simulink model "zynqRadioHWSWQPSKAD9361AD9364SL"  (R2025a)
settings: Solver=FixedStepDiscrete  StartTime=0.0  StopTime=0.5  RelTol=1e-3
PreLoadFcn:
  | setTxBurstLength = 10000;
  | txtmsg = ['Zynq radio HW/SW Co-design ÞÞÞÞ']; % Use only printable characters
  | 
  | %------------------------------------------------------------------------------------------------------
  | if ~isequal(size(txtmsg),[1 31])
  |     error('txtmsg must contain 31 characters');
  | end
  | 
  | [dataBits,msg] = zynqRadioHWSWQPSKgenHelloworldMsg(20); % generate 20 msgs for LUT
  | msgLUT = uint8(msg);
  | dataBitsLUT = dataBits(:);
  | Rsym                = 10e3;%1.92e6;
  | Config = zynqRadioHWSWQPSKTxRxParameters;
  | fs = Rsym*Config.SamplesPerSymbol;
  | word = [txtmsg newline];  % append a new line character to txtmsg
  | 
  | % The highest clock rate is 16 times the message character rate.
  | % As the message characters are fed at highest clock to FPGA
  | % repeat each character 16 times to maintain the message rate.
  | word = repelem(word.',16,1);
  | repeatTimes = ceil(setTxBurstLength/length(word));
  | inpData = complex(repmat(uint8(word),repeatTimes,1));
  | inUseTxBurstLength = length(inpData);
PostLoadFcn:
  | hScopeConfig = get_param([gcs '/HDL_QPSK/QPSK Tx Channel QPSK Rx/QPSK Rx/Frequency and Time Synchronizer/Symbol Synchronizer/No HDL/QPSK Receiver Eye Diagram'],'ScopeConfiguration');
  | hScopeConfig.OpenAtSimulationStart = false;
  | hScopeConfig.Visible = false;
  | clear hScopeConfig
InitFcn:
  | setTxBurstLength = 10000;
  | txtmsg = ['Zynq radio HW/SW Co-design ÞÞÞÞ']; % Use only printable characters
  | 
  | %------------------------------------------------------------------------------------------------------
  | if ~isequal(size(txtmsg),[1 31])
  |     error('txtmsg must contain 31 characters');
  | end
  | 
  | [dataBits,msg] = zynqRadioHWSWQPSKgenHelloworldMsg(20); % generate 20 msgs for LUT
  | msgLUT = uint8(msg);
  | dataBitsLUT = dataBits(:);
  | Rsym                = 10e3;%1.92e6;
  | Config = zynqRadioHWSWQPSKTxRxParameters;
  | fs = Rsym*Config.SamplesPerSymbol;
  | word = [txtmsg newline];  % append a new line character to txtmsg
  | 
  | % The highest clock rate is 16 times the message character rate.
  | % As the message characters are fed at highest clock to FPGA
  | % repeat each character 16 times to maintain the message rate.
  | word = repelem(word.',16,1);
  | repeatTimes = ceil(setTxBurstLength/length(word));
  | inpData = complex(repmat(uint8(word),repeatTimes,1));
  | inUseTxBurstLength = length(inpData);
  | 
  | Config.Preamble = logical(zeros(0,1))
undefined symbols (not defined in the file or in its folder): Add, dspblkCoreblockFVToolHelper, gcbh, gse_genframes, Shift
libraries: hdlsllib x144, simulink x37, dsphdlsigops2 x3, dsphdlfiltering2 x3, whdlutilities x3, dsphdlxfrm2 x2, dsphdlmathfun2 x2, commdigbbndpm3 x2, sdrzblksprivate x1
(part 3 of 6)

== system zynqRadioHWSWQPSKAD9361AD9364SL/HDL_QPSK/QPSK Tx Channel QPSK Rx/QPSK Rx/Frequency and Time Synchronizer/Symbol Synchronizer ==
  dataIn : Inport
  validIn : Inport  Port=2
  Data Type Conversion4 : DataTypeConversion  OutDataTypeStr=fixdt(1,16,14)  SaturateOnIntegerOverflow=off  RndMeth=Floor
  Delay{1..4,6,8..9} (7 alike) : Delay  DelayLength=1
  Delay5 : Delay  DelayLength=12
  Delay7 : Delay  DelayLength=12
  Gardner TED : Subsystem
  Integer Delay{1..4} (4 alike) : Delay  DelayLength=1
  Interpolation Control : MATLAB Function
  Interpolation Filter : Subsystem
  Loop Filter : Subsystem
  No HDL : Subsystem
  Rate Handle : Subsystem
  dataOut : Outport
  validOut : Outport  Port=2
  wires:
  Loop Filter/1(v) -> Delay4/1
  Gardner TED/1(e) -> Delay3/1
  Interpolation Control/2(Underflow) -> Integer Delay3/1
  Integer Delay4/1 -> Interpolation Filter/2(mu)
  dataIn/1 -> No HDL/1(data), Integer Delay1/1
  Integer Delay3/1 -> Delay5/1
  Delay3/1 -> Loop Filter/1(e)
  Delay4/1 -> Interpolation Control/1(Delta)
  Data Type Conversion4/1 -> Rate Handle/1(dataIn)
  Delay1/1 -> Data Type Conversion4/1
  Delay6/1 -> Rate Handle/3(validIn)
  Delay7/1 -> Delay6/1
  validIn/1 -> No HDL/2(valid), Integer Delay2/1
  Rate Handle/2(validOut) -> validOut/1
  Rate Handle/1(dataOut) -> dataOut/1
  Interpolation Filter/1(interpolant) -> Delay8/1, Delay1/1
  Interpolation Control/1(mu) -> Integer Delay4/1
  Delay2/1 -> Rate Handle/2(strobe)
  Delay5/1 -> Delay9/1, Delay2/1
  Integer Delay1/1 -> Interpolation Filter/1(In)
  Integer Delay2/1 -> Delay7/1
  Delay8/1 -> Gardner TED/1(data)
  Delay9/1 -> Gardner TED/2(strobe)

== system zynqRadioHWSWQPSKAD9361AD9364SL/HDL_QPSK/QPSK Tx Channel QPSK Rx/QPSK Rx/QPSK Demodulator/Serializer ==
  u : Inport
  In2 : Inport  Port=2
  Delay1 : Delay  DelayLength=1
  Delay4 : Delay  DelayLength=1
  Demux : Demux  Outputs=2
  HDL Counter : hdlsllib/Sources/HDL Counter  CountType=Count limited  CountInit=0  CountStep=1  CountMax=1  CountFromType=Initial value  CountFrom=0  CountResetPort=off  CountLoadPort=off  CountEnbPort=on  CountDirPort=off  CountHitOutputPort=off  CountDataType=Unsigned  CountWordLen=1  CountFracLen=0  CountSampTime=1
  Logical Operator : Logic  Operator=OR  AllPortsSameDT=off  OutDataTypeStr=boolean
  Multiport Switch : MultiPortSwitch  DataPortOrder=Zero-based contiguous  Inputs=2  zeroidx=on  SaturateOnIntegerOverflow=off  InputSameDT=off
  Unit Delay Enabled Synchronous : hdlsllib/Discrete/Unit Delay Enabled Synchronous  InitialCondition=0.0  SampleTime=-1
  Out1 : Outport
  Out2 : Outport  Port=2
  wires:
  Demux/2 -> Multiport Switch/3
  Logical Operator/1 -> Out2/1, HDL Counter/1
  In2/1 -> Unit Delay Enabled Synchronous/2, Delay1/1
  HDL Counter/1 -> Multiport Switch/1
  Delay4/1 -> Logical Operator/2
  u/1 -> Unit Delay Enabled Synchronous/1
  Multiport Switch/1 -> Out1/1
  Demux/1 -> Multiport Switch/2
  Delay1/1 -> Logical Operator/1, Delay4/1
  Unit Delay Enabled Synchronous/1 -> Demux/1

== system zynqRadioHWSWQPSKAD9361AD9364SL/HDL_QPSK/QPSK Tx Channel QPSK Rx/QPSK Tx/Bit Packetizer/Data Bits FIFO ==
  data : Inport
  push : Inport  Port=2
  Compare To Constant : simulink/Logic and Bit Operations/Compare To Constant  relop=>=  const=length(Preamble)  OutDataTypeStr=boolean
  Compare To Constant1 : simulink/Logic and Bit Operations/Compare To Constant  relop===  const=0  OutDataTypeStr=boolean
  Compare To Constant2 : simulink/Logic and Bit Operations/Compare To Constant  relop=~=  const=0  OutDataTypeStr=boolean
  Compare To Constant3 : simulink/Logic and Bit Operations/Compare To Constant  relop===  const=0  OutDataTypeStr=boolean
  Compare To Constant4 : simulink/Logic and Bit Operations/Compare To Constant  relop===  const=bitsPerPacket - 1  OutDataTypeStr=boolean
  Compare To Constant5 : hdlsllib/Logic and Bit Operations/Compare To Constant  relop===  const=Config.SamplesPerSymbol/2 -1  OutDataTypeStr=boolean
  Constant : Constant  Value=true  SampleTime=1/(Rsym*4)
  Delay{1..7} (7 alike) : Delay  DelayLength=1
  HDL Counter : hdlsllib/Sources/HDL Counter  CountType=Count limited  CountInit=0  CountStep=1  CountMax=dataBitsPerPacket*2 - 1  CountFromType=Initial value  CountFrom=0  CountResetPort=off  CountLoadPort=off  CountEnbPort=on  CountDirPort=off  CountHitOutputPort=off  CountDataType=Unsigned  CountWordLen=nextpow2(dataBitsPerPacket*2 - 1)  CountFracLen=0  CountSampTime=1
  HDL Counter1 : hdlsllib/Sources/HDL Counter  CountType=Count limited  CountInit=0  CountStep=1  CountMax=dataBitsPerPacket*2 - 1  CountFromType=Initial value  CountFrom=0  CountResetPort=off  CountLoadPort=off  CountEnbPort=on  CountDirPort=off  CountHitOutputPort=off  CountDataType=Unsigned  CountWordLen=nextpow2(dataBitsPerPacket*2 - 1)  CountFracLen=0  CountSampTime=1
  HDL Counter2 : hdlsllib/Sources/HDL Counter  CountType=Count limited  CountInit=0  CountStep=1  CountMax=bitsPerPacket - 1  CountFromType=Initial value  CountFrom=0  CountResetPort=off  CountLoadPort=off  CountEnbPort=on  CountDirPort=off  CountHitOutputPort=off  CountDataType=Unsigned  CountWordLen=nextpow2(bitsPerPacket)  CountFracLen=0  CountSampTime=1
  HDL Counter3 : hdlsllib/Sources/HDL Counter  CountType=Count limited  CountInit=0  CountStep=1  CountMax=Config.SamplesPerSymbol/2 -1  CountFromType=Initial value  CountFrom=0  CountResetPort=off  CountLoadPort=off  CountEnbPort=on  CountDirPort=off  CountHitOutputPort=off  CountDataType=Unsigned  CountWordLen=nextpow2(Config.SamplesPerSymbol/2)  CountFracLen=0  CountSampTime=1
  Logical Operator : Logic  Inputs=3  AllPortsSameDT=off  OutDataTypeStr=boolean
  Logical Operator1 : Logic  Inputs=3  AllPortsSameDT=off  OutDataTypeStr=boolean
  MATLAB Function1 : MATLAB Function  TreatAsAtomicUnit=on
  No HDL : Subsystem
  RAM Frame Status Indicator : MATLAB Function  TreatAsAtomicUnit=on
  Simple Dual Port RAM : hdlsllib/HDL RAMs/Simple Dual Port RAM  ram_size=nextpow2(dataBitsPerPacket*2 - 1)
  Unit Delay Enabled Resettable Synchronous : hdlsllib/Discrete/Unit Delay Enabled Resettable Synchronous  InitialCondition=0.0  SampleTime=-1
  dataOut : Outport
  activeFrame : Outport  Port=2
  sampleCount : Outport  Port=3
  sampleCountValid : Outport  Port=4
  fullRAM : Outport  Port=5
  wires:
  HDL Counter1/1 -> Simple Dual Port RAM/4
  HDL Counter/1 -> Simple Dual Port RAM/2
  data/1 -> Simple Dual Port RAM/1
  Constant/1 -> HDL Counter3/1
  HDL Counter2/1 -> Compare To Constant/1, Delay2/1, Compare To Constant3/1
  Compare To Constant1/1 -> Unit Delay Enabled Resettable Synchronous/3
  RAM Frame Status Indicator/1(out) -> Delay3/1
  Compare To Constant2/1 -> Logical Operator1/1, Unit Delay Enabled Resettable Synchronous/1
  Compare To Constant3/1 -> Unit Delay Enabled Resettable Synchronous/2
  Compare To Constant/1 -> Delay1/1
  Delay1/1 -> Logical Operator/2
  Delay2/1 -> Delay5/1
  Delay3/1 -> Compare To Constant2/1, Compare To Constant1/1
  Simple Dual Port RAM/1 -> dataOut/1
  Delay4/1 -> Logical Operator/3, Delay6/1
  Delay5/1 -> Compare To Constant4/1, sampleCount/1
  Delay6/1 -> Logical Operator1/3, sampleCountValid/1
  Unit Delay Enabled Resettable Synchronous/1 -> Logical Operator/1
  Compare To Constant4/1 -> Logical Operator1/2
  Logical Operator1/1 -> activeFrame/1
  Logical Operator/1 -> RAM Frame Status Indicator/2(pop), MATLAB Function1/2(rd), No HDL/2(pop), HDL Counter1/1
  push/1 -> MATLAB Function1/1(wr), RAM Frame Status Indicator/1(push), No HDL/1(push), HDL Counter/1, Simple Dual Port RAM/3
  MATLAB Function1/1(full) -> Delay7/1
  Delay7/1 -> fullRAM/1
  HDL Counter3/1 -> Compare To Constant5/1
  Compare To Constant5/1 -> HDL Counter2/1, Delay4/1

== system zynqRadioHWSWQPSKAD9361AD9364SL/HDL_QPSK/QPSK Tx Channel QPSK Rx/QPSK Tx/Bit Packetizer/Preamble Bits Generator ==
  activeFrame : Inport
  sampleCount : Inport  Port=2
  sampleCountValid : Inport  Port=3
  Compare To Constant2 : hdlsllib/Logic and Bit Operations/Compare To Constant  relop===  const=bitsPerPacket - 1  OutDataTypeStr=boolean
  Logical Operator3 : Logic  AllPortsSameDT=off  OutDataTypeStr=boolean
  Preamble Bits Store : Subsystem
  Unit Delay Enabled Synchronous : hdlsllib/Discrete/Unit Delay Enabled Synchronous  InitialCondition=0.0  SampleTime=-1
  preambleBits : Outport
  wires:
  sampleCount/1 -> Compare To Constant2/1, Preamble Bits Store/2(sampleCount)
  Logical Operator3/1 -> Unit Delay Enabled Synchronous/2
  Preamble Bits Store/1(preamble) -> preambleBits/1
  Compare To Constant2/1 -> Logical Operator3/1
  Unit Delay Enabled Synchronous/1 -> Preamble Bits Store/1(actualPreamble)
  sampleCountValid/1 -> Logical Operator3/2
  activeFrame/1 -> Unit Delay Enabled Synchronous/1

== system zynqRadioHWSWQPSKAD9361AD9364SL/HDL_QPSK/QPSK Tx Channel QPSK Rx/QPSK Tx/FEC Encoder/DVB-S2 BCH Encoder ==
  dataIn : Inport
  startIn : Inport  Port=2
  endIn : Inport  Port=3
  validIn : Inport  Port=4
  frameType : Inport  Port=5
  codeRateIdx : Inport  Port=6
  Input controller : Subsystem
  Output Controller : Subsystem
  Parity Generation : Subsystem
  Store and Retreive Input : Subsystem
  Terminator : Terminator
  dataOut : Outport
  ctrlOut : Outport  Port=2
  wires:
  Store and Retreive Input/2(outrd_data) -> Parity Generation/1(outrd_data)
  Store and Retreive Input/3(outRd_valid) -> Parity Generation/2(outRd_valid)
  Output Controller/1(outData) -> dataOut/1
  Output Controller/2(outCtrl) -> ctrlOut/1
  Store and Retreive Input/4(ParityCalCompFlag) -> Parity Generation/3(ParityCalCompFlag)
  Parity Generation/3(parityScalarOut) -> Output Controller/4(outputParity)
  Parity Generation/4(parityScalarValidOut) -> Output Controller/5(validParity)
  Output Controller/3(nxtFrame) -> Terminator/1
  Input controller/6(reset) -> Store and Retreive Input/7(resetIn)
  frameType/1 -> Input controller/4(frameType)
  codeRateIdx/1 -> Input controller/5(codeRateIdx)
  Input controller/1(iwr_enb) -> Store and Retreive Input/2(iwr_enb)
  Input controller/8(sampledStartIn) -> Output Controller/8(sampledStartIn)
  Input controller/2(iwr_addr) -> Store and Retreive Input/3(iwr_addr)
  Input controller/5(framLenDelayed) -> Store and Retreive Input/6(framLenDelayed)
  Input controller/3(ird_addr) -> Store and Retreive Input/4(ird_addr)
  Input controller/7(parLen) -> Output Controller/7(parLen), Parity Generation/5(parLen)
  Input controller/4(ird_valid) -> Store and Retreive Input/5(ird_valid)
  Input controller/11(frameLen) -> Output Controller/11(frameLen)
  Input controller/12(validCodeRate) -> Output Controller/12(validCodeRate)
  Input controller/13(unitFrameLen) -> Output Controller/13(unitFrameLen)
  dataIn/1 -> Store and Retreive Input/1(iwr_data)
  Store and Retreive Input/5(resetOut) -> Parity Generation/4(resetIn)
  Parity Generation/5(resetOut) -> Output Controller/6(resetIn)
  Parity Generation/1(readDataOut) -> Output Controller/2(outputMsg)
  Parity Generation/2(readValidOut) -> Output Controller/3(validMsg)
  Store and Retreive Input/1(framLenDelay) -> Output Controller/1(framLenDelayed)
  Input controller/9(enbBCHEnc) -> Output Controller/9(enbBCHEnc)
  Input controller/10(sampledEndIn) -> Output Controller/10(sampledEndIn)
  startIn/1 -> Input controller/1(startIn)
  endIn/1 -> Input controller/2(endIn)
  validIn/1 -> Input controller/3(validIn)

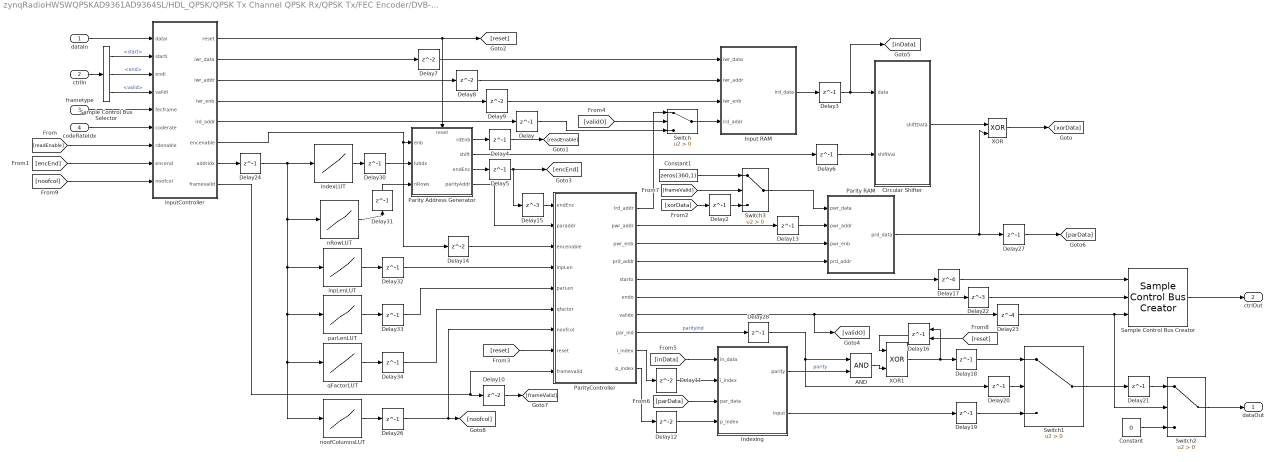
== system zynqRadioHWSWQPSKAD9361AD9364SL/HDL_QPSK/QPSK Tx Channel QPSK Rx/QPSK Tx/FEC Encoder/DVB-S2 LDPC Encoder ==
  dataIn : Inport
  ctrlIn : Inport  Port=2
  frametype : Inport  Port=3
  codeRateIdx : Inport  Port=4
  AND : Logic  IconShape=distinctive  AllPortsSameDT=off  OutDataTypeStr=boolean
  Circular Shifter : Subsystem
  Constant : Constant  Value=0  OutDataTypeStr=boolean  SampleTime=-1
  Constant1 : Constant  Value=zeros(360,1)  OutDataTypeStr=boolean  SampleTime=-1
  Delay{,2..6,13,18..21,24,26..28,30..34} (20 alike) : Delay  DelayLength=1
  Delay{7..10,14} (5 alike) : Delay
  Delay11 : Delay  InitialCondition=1
  Delay12 : Delay  InitialCondition=1
  Delay15 : Delay  DelayLength=3
  Delay16 : Delay  DelayLength=1  ExternalReset=Level
      settings: InputPortMap=u0,r5
  Delay17 : Delay  DelayLength=4
  Delay22 : Delay  DelayLength=3
  Delay23 : Delay  DelayLength=4  InitialCondition=0
  Indexing : MATLAB Function  TreatAsAtomicUnit=on
  Input RAM : Subsystem  TreatAsAtomicUnit=on
  Parity Address Generator : Subsystem
      settings: PortSchema="{\"entries\":[{\"content\":{\"sides\":[{\"content\":{\"connectorIds\":[\"In1\",\"In2\",\"In3\"]},\"type\":\"ConnectorPlacement.EquallySpacedRectSide\",\"uuid\":\"9edb1342-d6f5-499c-9bf1-f44ee53486a4\"},{\"content\":{\"connectorIds\":[\"Out1\",\"Out2\",\"Out3\",\"Out4\"],\"side\":\"RIGHT\"},\"type\":\"ConnectorPlacement.EquallySpacedRectSide\",\"uuid\":\"a3ac1c1a-65e5-420b-9f9b-56e74b10dc22\"},{\"content\":{\"connectorIds\":[\"In4\"],\"side\":\"TOP\"},\"type\":\"ConnectorPlacement.EquallySpacedRectSide\",\"uuid\":\"45c2534c-7de7-4c56-9dba-21058b31a7ef\"}]},\"type\":\"ConnectorPlacement.EquallySpacedConnector\",\"uuid\":\"218608a7-7b04-46f4-8613-c36872134e11\"}],\"packageUris\":[\"http://schema.mathworks.com/mf0/Connector/R2020b\"],\"version\":\"1.0\"}"
  Parity RAM : Subsystem  TreatAsAtomicUnit=on
  ParityController : MATLAB Function  TreatAsAtomicUnit=on
  Sample Control Bus Creator : whdlutilities/Sample Control Bus Creator
  Sample Control Bus Selector : whdlutilities/Sample Control Bus Selector  OutputSignals=start,end,valid
  Switch{,1..3} (4 alike) : Switch  Criteria=u2 > Threshold  SaturateOnIntegerOverflow=off  InputSameDT=off
  XOR : Logic  Operator=XOR  IconShape=distinctive  AllPortsSameDT=off  OutDataTypeStr=boolean
  XOR1 : Logic  Operator=XOR  IconShape=distinctive  AllPortsSameDT=off  OutDataTypeStr=fixdt(0,1,0)
  indexLUT : Lookup_n-D  NumberOfTableDimensions=1  BreakpointsSpecification=Even spacing  BreakpointsForDimension1=[1:20]  BreakpointsForDimension1FirstPoint=0  Table=[0,45,105,177,267,375,495,630,774,924,1084,1246,1246,1246,1246,1246,1246,1255,1270,1288,1308,1335,1365,1398,1433,1470,1510,1510,1510,1510,1510,1510]  InterpMethod=Flat  RemoveProtectionInput=on  InternalRulePriority=Speed  OutDataTypeStr=fixdt(0,11,0)  RndMeth=Simplest
  inpLenLUT : Lookup_n-D  NumberOfTableDimensions=1  BreakpointsSpecification=Even spacing  BreakpointsForDimension1=[1:20]  BreakpointsForDimension1FirstPoint=0  Table=[16200,21600,25920,32400,38880,43200,48600,51840,54000,57600,58320,58320,58320,58320,58320,58320,3240,5400,6480,7200,9720,10800,11880,12600,13320,14400,14400,14400,14400,14400,14400,14400]  InterpMethod=Flat  RemoveProtectionInput=on  InternalRulePriority=Speed  OutDataTypeStr=fixdt(0,16,0)  RndMeth=Simplest
  inputController : MATLAB Function  TreatAsAtomicUnit=on
  nRowLUT : Lookup_n-D  NumberOfTableDimensions=1  BreakpointsSpecification=Even spacing  BreakpointsForDimension1=[1:20]  BreakpointsForDimension1FirstPoint=0  Table=[45,60,72,90,108,120,135,144,150,160,162,162,162,162,162,162,9,15,18,20,27,30,33,35,37,40,40,40,40,40,40,40]  InterpMethod=Flat  RemoveProtectionInput=on  InternalRulePriority=Speed  OutDataTypeStr=fixdt(0,8,0)  RndMeth=Simplest
  noofColumnsLUT : Lookup_n-D  NumberOfTableDimensions=1  BreakpointsSpecification=Even spacing  BreakpointsForDimension1=[1:20]  BreakpointsForDimension1FirstPoint=0  Table=[45,60,72,90,108,120,135,144,150,160,162,162,162,162,162,162,9,15,18,20,27,30,33,35,37,40,40,40,40,40,40,40]  InterpMethod=Flat  RemoveProtectionInput=on  InternalRulePriority=Speed  OutDataTypeStr=uint8  RndMeth=Simplest
  parLenLUT : Lookup_n-D  NumberOfTableDimensions=1  BreakpointsSpecification=Even spacing  BreakpointsForDimension1=[1:20]  BreakpointsForDimension1FirstPoint=0  Table=[48600,43200,38880,32400,25920,21600,16200,12960,10800,7200,6480,6480,6480,6480,6480,6480,12960,10800,9720,9000,6480,5400,4320,3600,2880,1800,1800,1800,1800,1800,1800,1800]  InterpMethod=Flat  RemoveProtectionInput=on  InternalRulePriority=Speed  OutDataTypeStr=fixdt(0,16,0)  RndMeth=Simplest
  qFactorLUT : Lookup_n-D  NumberOfTableDimensions=1  BreakpointsSpecification=Even spacing  BreakpointsForDimension1=[1:20]  BreakpointsForDimension1FirstPoint=0  Table=[135,120,108,90,72,60,45,36,30,20,18,18,18,18,18,18,36,30,27,25,18,15,12,10,8,5,5,5,5,5,5,5]  InterpMethod=Flat  RemoveProtectionInput=on  InternalRulePriority=Speed  OutDataTypeStr=fixdt(0,9,0)  RndMeth=Simplest
  dataOut : Outport
  ctrlOut : Outport  Port=2
  wires:
  Delay6/1 -> Circular Shifter/2(shiftVal)
  Delay3/1 -> Circular Shifter/1(data), [inData]
  Delay28/1 -> AND/1, Delay20/1
  Delay27/1 -> [parData]
  Input RAM/1(ird_data) -> Delay3/1
  Delay22/1 -> Sample Control Bus Creator/2
  Parity RAM/1(prd_data) -> XOR/2, Delay27/1
  [validO] -> Switch/2
  [noofcol] -> inputController/9(noofcol)
  Delay26/1 -> [noofcol], ParityController/7(noofcol)
  noofColumnsLUT/1 -> Delay26/1
  ParityController/7(valido) -> Delay23/1, [validO]
  Delay34/1 -> ParityController/6(qfactor)
  Delay33/1 -> ParityController/5(parLen)
  Delay32/1 -> ParityController/4(inpLen)
  Delay31/1 -> Parity Address Generator/3(nRows)
  Delay30/1 -> Parity Address Generator/2(lutIdx)
  ParityController/5(starto) -> Delay17/1
  ParityController/10(p_index) -> Delay12/1
  ParityController/1(ird_addr) -> Switch/1
  ParityController/4(prd_addr) -> Parity RAM/4(prd_addr)
  Circular Shifter/1(shiftData) -> XOR/1
  Sample Control Bus Selector/3 -> inputController/4(validi)  "<valid>"
  [inData] -> Indexing/1(in_data)
  Delay18/1 -> Switch1/1
  indexLUT/1 -> Delay30/1
  Delay5/1 -> Delay15/1, [encEnd]
  XOR/1 -> [xorData]
  inputController/8(framevalid) -> ParityController/9(framevalid), Delay10/1
  Delay16/1 -> XOR1/1
  Delay13/1 -> Parity RAM/2(pwr_addr)
  inputController/2(iwr_data) -> Delay7/1
  ParityController/8(par_ind) -> Delay28/1  "parityInd"
  Delay14/1 -> ParityController/3(encenable)
  Delay8/1 -> Input RAM/2(iwr_addr)
  inputController/5(ird_addr) -> Delay/1
  Delay23/1 -> Switch2/2, Sample Control Bus Creator/3
  inpLenLUT/1 -> Delay32/1
  Constant/1 -> Switch2/3
  Switch/1 -> Input RAM/4(ird_addr)
  Sample Control Bus Selector/2 -> inputController/3(endi)  "<end>"
  Delay2/1 -> Switch3/3
  [reset] -> Delay16/2
  Sample Control Bus Creator/1 -> ctrlOut/1
  Constant1/1 -> Switch3/1
  ctrlIn/1 -> Sample Control Bus Selector/1
  codeRateIdx/1 -> inputController/6(coderate)
  frametype/1 -> inputController/5(fecframe)
  dataIn/1 -> inputController/1(datai)
  inputController/3(iwr_addr) -> Delay8/1
  Sample Control Bus Selector/1 -> inputController/2(starti)  "<start>"
  Switch3/1 -> Parity RAM/1(pwr_data)
  [frameValid] -> Switch3/2
  Delay17/1 -> Sample Control Bus Creator/1
  Switch1/1 -> Delay21/1
  [xorData] -> Delay2/1
  Delay11/1 -> Indexing/2(i_index)
  Delay12/1 -> Indexing/4(p_index)
  Delay9/1 -> Input RAM/3(iwr_enb)
  Parity Address Generator/2(shift) -> Delay6/1
  Delay24/1 -> indexLUT/1, nRowLUT/1, inpLenLUT/1, parLenLUT/1, qFactorLUT/1, noofColumnsLUT/1
  [readEnable] -> inputController/7(rdenable)
  Parity Address Generator/1(rdEnb) -> Delay4/1
  AND/1 -> XOR1/2
  Delay21/1 -> Switch2/1
  [parData] -> Indexing/3(par_data)
  qFactorLUT/1 -> Delay34/1
  Parity Address Generator/4(parityAddr) -> ParityController/2(paraddr)
  inputController/7(addridx) -> Delay24/1
  [encEnd] -> inputController/8(encend)
  Delay19/1 -> Switch1/3
  nRowLUT/1 -> Delay31/1
  inputController/6(encenable) -> Delay14/1, Parity Address Generator/1(enb)
  inputController/1(reset) -> [reset], Parity Address Generator/4(reset)
  Delay/1 -> Switch/3
  parLenLUT/1 -> Delay33/1
  Delay4/1 -> [readEnable]
  Delay15/1 -> ParityController/1(endEnc)
  Delay20/1 -> Switch1/2
  ParityController/3(pwr_enb) -> Parity RAM/3(pwr_enb)
  Delay10/1 -> [frameValid]
  ParityController/6(endo) -> Delay22/1
  Delay7/1 -> Input RAM/1(iwr_data)
  inputController/4(iwr_enb) -> Delay9/1
  Indexing/1(parity) -> AND/2  "parity"
  [reset] -> ParityController/8(reset)
  Indexing/2(input) -> Delay19/1
  XOR1/1 -> Delay18/1, Delay16/1
  Parity Address Generator/3(endEnc) -> Delay5/1
  Switch2/1 -> dataOut/1
  ParityController/9(i_index) -> Delay11/1
  ParityController/2(pwr_addr) -> Delay13/1

== system zynqRadioHWSWQPSKAD9361AD9364SL/HDL_QPSK/QPSK Tx Channel QPSK Rx/QPSK Rx/Frequency and Time Synchronizer/Carrier Synchronizer/Direct Digital Synthesis ==
  rst : Inport
  validIn : Inport  Port=2
  phaseInc : Inport  Port=3
  Data Type Conversion : DataTypeConversion  OutDataTypeStr=fixdt(1,21,21)  SaturateOnIntegerOverflow=off  RndMeth=Floor
  Data Type Conversion1 : DataTypeConversion  OutDataTypeStr=fixdt(1,21,0)  ConvertRealWorld=Stored Integer (SI)  SaturateOnIntegerOverflow=off  RndMeth=Floor
  Delay : Delay  DelayLength=1
  NCO : dsphdlsigops2/NCO  PhaseIncrementSource=Input port  PhaseIncrement=0  PhaseOffsetSource=Property  PhaseOffset=0  DitherSource=Property  NumDitherBits=11  SamplesPerFrame=1  LUTCompress=off  ResetAction=on  Waveform=Complex exponential  PhasePort=off  SimulateUsing=Code generation  AccumulatorWL=21  PhaseQuantization=on  NumQuantizerAccumulatorBits=14  OutputDataType=Binary point scaling  OutputWL=16  OutputFL=14
  Terminator : Terminator
  expOut : Outport
  wires:
  Data Type Conversion/1 -> Data Type Conversion1/1
  NCO/1 -> expOut/1
  validIn/1 -> NCO/3
  Data Type Conversion1/1 -> NCO/1
  NCO/2 -> Terminator/1
  Delay/1 -> Data Type Conversion/1
  phaseInc/1 -> Delay/1
  rst/1 -> NCO/2

== system zynqRadioHWSWQPSKAD9361AD9364SL/HDL_QPSK/QPSK Tx Channel QPSK Rx/QPSK Rx/Frequency and Time Synchronizer/Carrier Synchronizer/Loop Filter ==
  e : Inport
  validIn : Inport  Port=2
  internalRst : Inport  Port=3
  externalRst : Inport  Port=4
  Add : Sum  Inputs=+|+
  Add1 : Sum  Inputs=|++  OutDataTypeStr=Inherit: Same as first input
  Data Type Conversion1 : DataTypeConversion  OutDataTypeStr=fixdt(1,29,29)  SaturateOnIntegerOverflow=off  RndMeth=Floor
  Data Type Conversion2 : DataTypeConversion  OutDataTypeStr=fixdt(1,39,39)  SaturateOnIntegerOverflow=off  RndMeth=Floor
  Delay : Delay  DelayLength=1
  Delay{1..11,13} (12 alike) : Delay
  Delay12 : Delay  DelayLength=1
  Gain : Gain  Gain=fi(CSLoopFilterIntegGain/(2*pi),0,16,16)  ParamDataTypeStr=Inherit: Inherit from 'Gain'
  Gain1 : Gain  Gain=fi(CSLoopFilterPropGain/(2*pi),0,16,16)  ParamDataTypeStr=Inherit: Inherit from 'Gain'
  Logical Operator : Logic  Operator=OR  AllPortsSameDT=off  OutDataTypeStr=boolean
  Unit Delay Enabled Resettable Synchronous : hdlsllib/Discrete/Unit Delay Enabled Resettable Synchronous  InitialCondition=0.0  SampleTime=-1
  Unit Delay Enabled Resettable Synchronous1 : hdlsllib/Discrete/Unit Delay Enabled Resettable Synchronous  InitialCondition=0.0  SampleTime=-1
  v : Outport
  valid : Outport  Port=2
  rst : Outport  Port=3
  wires:
  Delay6/1 -> Data Type Conversion1/1
  Delay5/1 -> Gain/1
  Delay7/1 -> Gain1/1
  Gain/1 -> Delay1/1
  Data Type Conversion2/1 -> Add1/1
  Delay3/1 -> Add/2
  Delay1/1 -> Data Type Conversion2/1
  Gain1/1 -> Delay6/1
  Delay2/1 -> Add/1
  Add/1 -> v/1
  e/1 -> Delay7/1, Delay5/1
  Data Type Conversion1/1 -> Unit Delay Enabled Resettable Synchronous/1
  Add1/1 -> Unit Delay Enabled Resettable Synchronous1/1
  Unit Delay Enabled Resettable Synchronous1/1 -> Delay3/1, Add1/2
  Unit Delay Enabled Resettable Synchronous/1 -> Delay2/1
  Logical Operator/1 -> Unit Delay Enabled Resettable Synchronous/3, Unit Delay Enabled Resettable Synchronous1/3
  validIn/1 -> Delay8/1
  Delay8/1 -> Delay4/1
  externalRst/1 -> Logical Operator/1
  internalRst/1 -> Delay9/1
  Delay9/1 -> Delay10/1
  Delay10/1 -> Delay12/1, Logical Operator/2
  Delay4/1 -> Unit Delay Enabled Resettable Synchronous/2, Unit Delay Enabled Resettable Synchronous1/2, Delay/1
  Delay11/1 -> valid/1
  Delay/1 -> Delay11/1
  Delay12/1 -> Delay13/1
  Delay13/1 -> rst/1

== system zynqRadioHWSWQPSKAD9361AD9364SL/HDL_QPSK/QPSK Tx Channel QPSK Rx/QPSK Rx/Frequency and Time Synchronizer/Carrier Synchronizer/Phase Error Detector ==
  dataIn : Inport
  Add : Sum  Inputs=+|-
  Compare To Constant : simulink/Logic and Bit Operations/Compare To Constant  relop=>=  const=0  OutDataTypeStr=boolean
  Compare To Constant1 : simulink/Logic and Bit Operations/Compare To Constant  relop=>=  const=0  OutDataTypeStr=boolean
  Complex to Real-Imag : ComplexToRealImag
  Constant : Constant  OutDataTypeStr=fixdt(1,2,0)  SampleTime=1/(Rsym*SamplesPerSymbol)
  Constant1 : Constant  Value=-1  OutDataTypeStr=fixdt(1,2,0)  SampleTime=1/(Rsym*SamplesPerSymbol)
  Constant2 : Constant  OutDataTypeStr=fixdt(1,2,0)  SampleTime=1/(Rsym*SamplesPerSymbol)
  Constant3 : Constant  Value=-1  OutDataTypeStr=fixdt(1,2,0)  SampleTime=1/(Rsym*SamplesPerSymbol)
  Data Type Conversion3 : DataTypeConversion  OutDataTypeStr=fixdt(1,10+3,10)  SaturateOnIntegerOverflow=off  RndMeth=Floor
  Delay{,1..6} (7 alike) : Delay
  Product : Product
  Product1 : Product
  Switch : Switch  Threshold=1  SaturateOnIntegerOverflow=off  InputSameDT=off
  Switch1 : Switch  Threshold=1  SaturateOnIntegerOverflow=off  InputSameDT=off
  PhaseError : Outport
  wires:
  Complex to Real-Imag/1 -> Delay2/1, Compare To Constant/1
  Compare To Constant1/1 -> Switch1/2
  Constant/1 -> Switch/1
  Constant3/1 -> Switch1/3
  Constant2/1 -> Switch1/1
  Constant1/1 -> Switch/3
  Compare To Constant/1 -> Switch/2
  Add/1 -> Delay6/1
  Switch/1 -> Delay/1
  Product1/1 -> Delay5/1
  Product/1 -> Delay4/1
  Switch1/1 -> Delay3/1
  Complex to Real-Imag/2 -> Delay1/1, Compare To Constant1/1
  dataIn/1 -> Complex to Real-Imag/1
  Delay/1 -> Product/1
  Delay1/1 -> Product/2
  Delay2/1 -> Product1/1
  Delay3/1 -> Product1/2
  Delay4/1 -> Add/1
  Delay5/1 -> Add/2
  Delay6/1 -> Data Type Conversion3/1
  Data Type Conversion3/1 -> PhaseError/1

== system zynqRadioHWSWQPSKAD9361AD9364SL/HDL_QPSK/QPSK Tx Channel QPSK Rx/QPSK Rx/Frequency and Time Synchronizer/Coarse Frequency Compensator/CFO step change detector ==
  note: fixed point precision loss warning supressed for this subsystem
  In1 : Inport
  Add : Sum  Inputs=+-
  Compare To Constant : simulink/Logic and Bit Operations/Compare To Constant  relop=>  const=CFOChangeDetectThreshold  OutDataTypeStr=boolean
  Compare To Constant1 : simulink/Logic and Bit Operations/Compare To Constant  relop=<  const=-CFOChangeDetectThreshold  OutDataTypeStr=boolean
  Delay : Delay  DelayLength=6
  Delay1 : Delay  DelayLength=1
  Logical Operator : Logic  Operator=OR  AllPortsSameDT=off  OutDataTypeStr=boolean
  Out1 : Outport
  wires:
  In1/1 -> Add/1, Delay1/1
  Delay/1 -> Out1/1
  Delay1/1 -> Add/2
  Add/1 -> Compare To Constant/1, Compare To Constant1/1
  Compare To Constant/1 -> Logical Operator/1
  Logical Operator/1 -> Delay/1
  Compare To Constant1/1 -> Logical Operator/2

== system zynqRadioHWSWQPSKAD9361AD9364SL/HDL_QPSK/QPSK Tx Channel QPSK Rx/QPSK Rx/Frequency and Time Synchronizer/Coarse Frequency Compensator/Coarse Frequency Estimator ==
  dataIn : Inport
  validIn : Inport  Port=2
  Delay{1,9..12} (5 alike) : Delay  DelayLength=1
  Delay{2..8} (7 alike) : Delay
  Extract Frequency : Subsystem
  Gain1 : Gain  Gain=1/integAvgLen  ParamDataTypeStr=fixdt(0,nextpow2(integAvgLen),nextpow2(integAvgLen))  OutDataTypeStr=Inherit: Same as input
  Integrator : Subsystem
  Math Function : Math  Operator=conj
  Product : Product
  Unit Delay Enabled Synchronous : hdlsllib/Discrete/Unit Delay Enabled Synchronous  InitialCondition=0.0  SampleTime=-1
  normFreqEst : Outport
  wires:
  Delay8/1 -> Product/2
  Delay7/1 -> Product/1
  Delay6/1 -> Delay3/1
  Delay4/1 -> Integrator/2(validIn)
  Delay2/1 -> Integrator/1(dataIn)
  Delay1/1 -> Delay7/1
  Unit Delay Enabled Synchronous/1 -> Delay12/1
  Delay9/1 -> Delay6/1
  Delay3/1 -> Delay4/1
  Delay5/1 -> Gain1/1
  Gain1/1 -> Delay2/1
  Product/1 -> Delay5/1
  Math Function/1 -> Delay8/1
  Delay10/1 -> Extract Frequency/1(datain)
  Delay11/1 -> Extract Frequency/2(validIn)
  Integrator/1(IntegOut) -> Delay10/1
  Integrator/2(IntegValid) -> Delay11/1
  Extract Frequency/1(normFreqOut) -> normFreqEst/1
  dataIn/1 -> Delay1/1, Unit Delay Enabled Synchronous/1
  validIn/1 -> Unit Delay Enabled Synchronous/2, Delay9/1
  Delay12/1 -> Math Function/1

== system zynqRadioHWSWQPSKAD9361AD9364SL/HDL_QPSK/QPSK Tx Channel QPSK Rx/QPSK Rx/Frequency and Time Synchronizer/Coarse Frequency Compensator/Raise Power to 4 ==
  dataIn : Inport
  validIn : Inport  Port=2
  Delay{1..8,11..12} (10 alike) : Delay
  Delay10 : Delay  DelayLength=1
  Delay9 : Delay  DelayLength=1
  Product1 : Product  OutDataTypeStr=Inherit: Same as first input
  Product2 : Product  OutDataTypeStr=Inherit: Same as first input
  dataOut : Outport
  validOut : Outport  Port=2
  wires:
  Delay12/1 -> validOut/1
  Delay11/1 -> dataOut/1
  Delay10/1 -> Delay8/1
  Delay9/1 -> Delay6/1, Delay7/1
  Delay8/1 -> Delay12/1
  Delay7/1 -> Product2/2
  Delay6/1 -> Product2/1
  Delay5/1 -> Delay2/1
  Delay4/1 -> Product1/2
  Delay3/1 -> Product1/1
  validIn/1 -> Delay5/1
  Product2/1 -> Delay11/1
  Delay2/1 -> Delay10/1
  Product1/1 -> Delay1/1
  Delay1/1 -> Delay9/1
  dataIn/1 -> Delay4/1, Delay3/1

== system zynqRadioHWSWQPSKAD9361AD9364SL/HDL_QPSK/QPSK Tx Channel QPSK Rx/QPSK Rx/Frequency and Time Synchronizer/No HDL/Subsystem ==
  In1 : Inport
  Enable : EnablePort
  To Workspace : ToWorkspace  VariableName=simAfterCS  SampleTime=-1
      settings: Save2DSignal=2-D array (concatenate along first dimension)
  wires:
  In1/1 -> To Workspace/1

== system zynqRadioHWSWQPSKAD9361AD9364SL/HDL_QPSK/QPSK Tx Channel QPSK Rx/QPSK Rx/Frequency and Time Synchronizer/Packet Controller/End Generator ==
  validIn : Inport
  rst : Inport  Port=2
  Compare To Constant : simulink/Logic and Bit Operations/Compare To Constant  relop===  const=1120-1  OutDataTypeStr=boolean
  Delay6 : Delay  DelayLength=1
  HDL Counter : hdlsllib/Sources/HDL Counter  CountType=Count limited  CountInit=0  CountStep=1  CountMax=1120 -1  CountFromType=Initial value  CountFrom=0  CountResetPort=on  CountLoadPort=off  CountEnbPort=on  CountDirPort=off  CountHitOutputPort=off  CountDataType=Unsigned  CountWordLen=nextpow2(1120-1)  CountFracLen=0  CountSampTime=1
  Logical Operator1 : Logic  IconShape=distinctive  AllPortsSameDT=off  OutDataTypeStr=boolean
  endOut : Outport
  wires:
  Compare To Constant/1 -> Logical Operator1/1
  HDL Counter/1 -> Compare To Constant/1
  validIn/1 -> HDL Counter/2, Logical Operator1/2
  rst/1 -> HDL Counter/1
  Logical Operator1/1 -> Delay6/1
  Delay6/1 -> endOut/1

== system zynqRadioHWSWQPSKAD9361AD9364SL/HDL_QPSK/QPSK Tx Channel QPSK Rx/QPSK Rx/Frequency and Time Synchronizer/Phase Ambiguity Estimation and Correction/Average Estimates ==
  endIn : Inport
  estin : Inport  Port=2
  validIn : Inport  Port=3
  Add : Sum  Inputs=++|
  Data Type Conversion : DataTypeConversion  OutDataTypeStr=fixdt(1,16+8,13)  SaturateOnIntegerOverflow=off  RndMeth=Floor
  Data Type Conversion1 : DataTypeConversion  OutDataTypeStr=fixdt(1,16+8,13)  SaturateOnIntegerOverflow=off  RndMeth=Floor
  Data Type Conversion2 : DataTypeConversion  OutDataTypeStr=fixdt(1,16,14)  SaturateOnIntegerOverflow=off  RndMeth=Floor
  Delay{,1..3} (4 alike) : Delay  DelayLength=1
  Divide by 8 : DataTypeConversion  OutDataTypeStr=fixdt(1,24,13+log2(8))  ConvertRealWorld=Stored Integer (SI)  SaturateOnIntegerOverflow=off  RndMeth=Floor
  Unit Delay Enabled Synchronous : hdlsllib/Discrete/Unit Delay Enabled Synchronous  InitialCondition=0.0  SampleTime=-1
  Unit Delay Enabled Resettable Synchronous : hdlsllib/Discrete/Unit Delay Enabled Resettable Synchronous  InitialCondition=0.0  SampleTime=-1
  avgEst : Outport
  wires:
  validIn/1 -> Delay1/1
  estin/1 -> Delay/1
  Data Type Conversion/1 -> Add/2
  Add/1 -> Data Type Conversion1/1
  Unit Delay Enabled Resettable Synchronous/1 -> Add/1, Divide by 8/1
  Data Type Conversion1/1 -> Unit Delay Enabled Resettable Synchronous/1
  Delay/1 -> Data Type Conversion/1
  Delay1/1 -> Unit Delay Enabled Resettable Synchronous/2
  endIn/1 -> Delay2/1
  Delay2/1 -> Delay3/1, Unit Delay Enabled Synchronous/2
  Delay3/1 -> Unit Delay Enabled Resettable Synchronous/3
  Divide by 8/1 -> Unit Delay Enabled Synchronous/1
  Unit Delay Enabled Synchronous/1 -> Data Type Conversion2/1
  Data Type Conversion2/1 -> avgEst/1

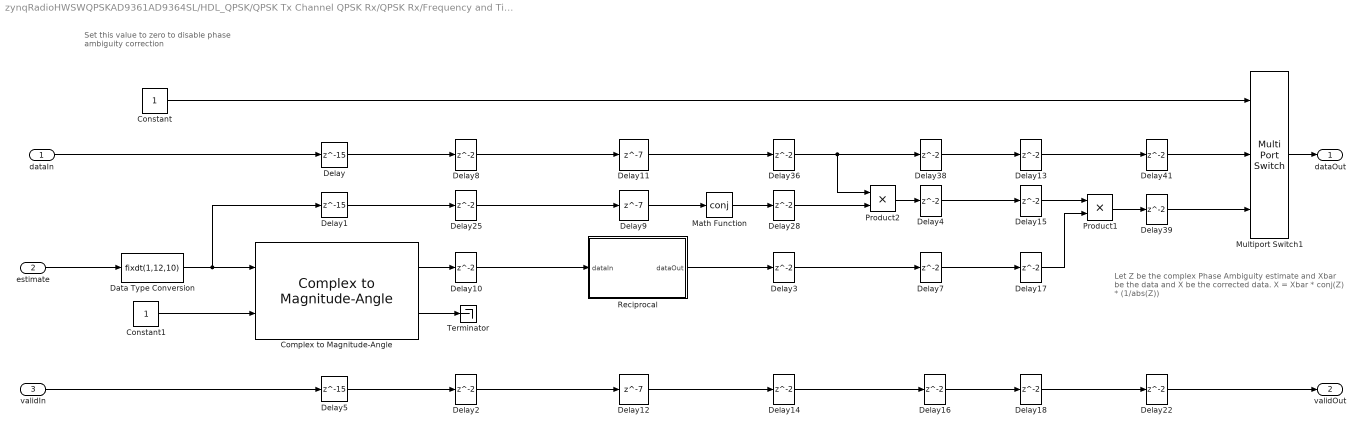
== system zynqRadioHWSWQPSKAD9361AD9364SL/HDL_QPSK/QPSK Tx Channel QPSK Rx/QPSK Rx/Frequency and Time Synchronizer/Phase Ambiguity Estimation and Correction/Phase Ambiguity Corrector ==
  note: Let Z be the complex Phase Ambiguity estimate and Xbar be the data and X be the corrected data.
      | X = Xbar * conj(Z) * (1/abs(Z))
  note: Set this value to zero to disable phase ambiguity correction
  dataIn : Inport
  estimate : Inport  Port=2
  validIn : Inport  Port=3
  Complex to Magnitude-Angle : dsphdlmathfun2/Complex to Magnitude-Angle  NumIterationsSource=Auto  NumIterations=10  OutputFormat=Magnitude  AngleFormat=Normalized  ScaleOutput=on  ScalingMethod=Shift-Add  SimulateUsing=Code generation
  Constant : Constant  OutDataTypeStr=boolean  SampleTime=-1
  Constant1 : Constant  OutMin=1  OutMax=1  OutDataTypeStr=boolean  SampleTime=-1
  Data Type Conversion : DataTypeConversion  OutDataTypeStr=fixdt(1,12,10)  SaturateOnIntegerOverflow=off  RndMeth=Floor
  Delay : Delay  DelayLength=15
  Delay1 : Delay  DelayLength=15
  Delay{2..4,7..8,10,13..18,22,25,28,36,38..39,41} (19 alike) : Delay  InitialCondition=0
  Delay11 : Delay  DelayLength=7  InitialCondition=0
  Delay12 : Delay  DelayLength=7  InitialCondition=0
  Delay5 : Delay  DelayLength=15
  Delay9 : Delay  DelayLength=7  InitialCondition=0
  Math Function : Math  Operator=conj  SignedPower=on  RndMeth=Zero
  Multiport Switch1 : MultiPortSwitch  DataPortOrder=Zero-based contiguous  Inputs=2  zeroidx=on  SaturateOnIntegerOverflow=off  InputSameDT=off
  Product1 : Product  OutDataTypeStr=Inherit: Same as first input
  Product2 : Product  OutDataTypeStr=Inherit: Same as first input
  Reciprocal : Subsystem  mask{WL=13, FL=10, outWL=26, Mapp=RAM - Based}
      mask prompts: WL "Input Word Length :"; FL "Input Fractional Length :"; outWL "Output Word Length :"; Mapp "Mapping Type:"
      mask init:
      | % Inverse for 18 bit numbers: partitioned into 3+15 bits. 2^3 LUTs with 2^15
      | % combinations will store a total of 2^18 combinations.
      | % As each LUT has 2^15 combinations the data type of output has a maximum
      | % limit of 32 bits (2^20 is a maximum number of bits an LUT can store)
      | 
      | % Non tunable Parameters
      | % FL = 16;
      | % outWL = 31;
      | % WL = 18;
      | % This Parameter is not given for mask
      | LUTAddrWL = WL - 1; % this will implement 2 LUTs
      | 
      | % validate Non tunable parameters
      | % condition for validation: 2^20 bits is the maximum number of bits an LUT can store
      | if LUTAddrWL >= 20   % As 2^20 is the limit
      |     error('invalid LUTAddrWL');
      | end
      | if outWL >= 2^(20-LUTAddrWL)  % 2^(20-LUTAddrWL) is the maximum outWL based on condition for validation
      |     error('invalid outWL')
      | end
      | 
      | % calculate number of LUTs required
      | muxSelectorWL = WL - LUTAddrWL;
      | nLUT = 2^muxSelectorWL;
      | 
      | % Generate all possible RWV inputs using WL and FL
      | allInputRangeSI = -2^(WL-1):2^(WL-1)-1;  % as a stored integer
      | allInputRWV = allInputRangeSI * 2^(-FL);
      | 
      | % define the function for all the RWV input
      | reciprocal = 1./allInputRWV;
      | 
      | % store the function output in LUT
      | allLUTAddr = (0:2^LUTAddrWL-1);
      | LUT = zeros(length(allLUTAddr),nLUT);
      | for i = 0:nLUT-1
      |     LUT(:,i+1) = reciprocal(i*2^LUTAddrWL+1:(i+1)*2^LUTAddrWL);
      | end
      | 
      | % quantize the function with outWL
      | NT = numerictype(fi(LUT(abs(LUT) ~= inf),1,outWL)); % inf and -inf will be quantized with max and min values with NT data type
      | if NT.WordLength < NT. FractionLength
      |     NT.FractionLength = NT.WordLength
      | end
      | LUT = fi(LUT,NT);
      | 
      | paths = find_system([gcb '/Function Impl'],'BlockType','Delay');
      | 
      | for i = 1:length(paths)
      |     if Mapp == 1
      |         hdlset_param(paths{i},'ResetType','default');
      |     else
      |         hdlset_param(paths{i},'ResetType','none');
      |     end
      | end
      mask TypeOptions Mapp: LUT - Based | RAM - Based
      mask DialogControl DescGroupVar Prompt: LUT - Based function
      mask DialogControl DescTextVar Prompt: This block is implemented for complex reciprocal
      mask Display: disp(['Reciprocal\n' get_param(gcb,'Mapp') '\nLatency = 7'])
  Terminator : Terminator
  dataOut : Outport
  validOut : Outport  Port=2
  wires:
  Delay3/1 -> Delay7/1
  Delay18/1 -> Delay22/1
  Delay17/1 -> Product1/2
  Delay15/1 -> Product1/1
  Delay13/1 -> Delay41/1
  Delay10/1 -> Reciprocal/1(dataIn)
  Delay12/1 -> Delay14/1
  Delay11/1 -> Delay36/1
  Delay9/1 -> Math Function/1
  Delay4/1 -> Delay15/1
  Delay41/1 -> Multiport Switch1/2
  Delay8/1 -> Delay11/1
  Delay/1 -> Delay8/1
  dataIn/1 -> Delay/1
  validIn/1 -> Delay5/1
  Delay5/1 -> Delay2/1
  Delay2/1 -> Delay12/1
  Delay14/1 -> Delay16/1
  Product2/1 -> Delay4/1
  Multiport Switch1/1 -> dataOut/1
  Delay22/1 -> validOut/1
  Constant/1 -> Multiport Switch1/1
  Delay16/1 -> Delay18/1
  Delay28/1 -> Product2/2
  Math Function/1 -> Delay28/1
  Delay25/1 -> Delay9/1
  Delay1/1 -> Delay25/1
  Delay36/1 -> Product2/1, Delay38/1
  Delay38/1 -> Delay13/1
  estimate/1 -> Data Type Conversion/1
  Reciprocal/1(dataOut) -> Delay3/1
  Product1/1 -> Delay39/1
  Constant1/1 -> Complex to Magnitude-Angle/2
  Complex to Magnitude-Angle/1 -> Delay10/1
  Complex to Magnitude-Angle/2 -> Terminator/1
  Delay39/1 -> Multiport Switch1/3
  Delay7/1 -> Delay17/1
  Data Type Conversion/1 -> Delay1/1, Complex to Magnitude-Angle/1

== system zynqRadioHWSWQPSKAD9361AD9364SL/HDL_QPSK/QPSK Tx Channel QPSK Rx/QPSK Rx/Frequency and Time Synchronizer/Phase Ambiguity Estimation and Correction/Phase Ambiguity Estimator ==
  dataIn : Inport
  syncPulse : Inport  Port=2
  validIn : Inport  Port=3
  Compare To Constant : simulink/Logic and Bit Operations/Compare To Constant  relop===  const=7  OutDataTypeStr=boolean
  Delay{1..3,8} (4 alike) : Delay  DelayLength=1
  Delay{4..7,9..11} (7 alike) : Delay
  Direct Lookup Table (n-D) : LookupNDDirect  NumberOfTableDimensions=1  Table=fi(preambleSymbols(3+1:3+8),1,16)  DiagnosticForOutOfRangeInput=Error
  HDL Counter : hdlsllib/Sources/HDL Counter  CountType=Count limited  CountInit=0  CountStep=1  CountMax=8-1  CountFromType=Initial value  CountFrom=0  CountResetPort=on  CountLoadPort=off  CountEnbPort=on  CountDirPort=off  CountHitOutputPort=off  CountDataType=Unsigned  CountWordLen=3  CountFracLen=0  CountSampTime=1
  Logical Operator : Logic  IconShape=distinctive  AllPortsSameDT=off  OutDataTypeStr=boolean
  Math Function : Math  Operator=conj  SignedPower=on  RndMeth=Zero
  Product : Product
  Subsystem : Subsystem
  Subsystem1 : Subsystem
  endOut : Outport
  estOut : Outport  Port=2
  validOut : Outport  Port=3
  wires:
  Compare To Constant/1 -> Logical Operator/2
  Subsystem/1(Out2) -> Subsystem1/1(In1), HDL Counter/1
  Direct Lookup Table (n-D)/1 -> Math Function/1
  Math Function/1 -> Delay4/1
  Product/1 -> Delay9/1
  Delay8/1 -> Direct Lookup Table (n-D)/1
  Delay1/1 -> Delay5/1
  Delay2/1 -> Delay6/1
  Delay3/1 -> Delay7/1
  Delay4/1 -> Product/2
  Delay5/1 -> Product/1
  Delay6/1 -> Delay10/1
  Delay7/1 -> Delay11/1
  Delay9/1 -> estOut/1
  Delay10/1 -> validOut/1
  Delay11/1 -> endOut/1
  dataIn/1 -> Delay1/1
  HDL Counter/1 -> Delay8/1, Compare To Constant/1
  Subsystem1/1(validOut) -> Delay2/1, Logical Operator/1, HDL Counter/2
  Logical Operator/1 -> Delay3/1, Subsystem/2(H)
  syncPulse/1 -> Subsystem/1(L)
  validIn/1 -> Subsystem1/2(validIn)

== system zynqRadioHWSWQPSKAD9361AD9364SL/HDL_QPSK/QPSK Tx Channel QPSK Rx/QPSK Rx/Frequency and Time Synchronizer/Preamble Detector/Correlator ==
  dataIn : Inport
  validIn : Inport  Port=2
  Complex to Real-Imag : ComplexToRealImag  Output=Real
  Delay{1..6} (6 alike) : Delay  DelayLength=1
  Delay7 : Delay  DelayLength=4
  Delay8 : Delay  DelayLength=4
  Discrete FIR Filter : dsphdlfiltering2/Discrete FIR Filter  NumeratorSource=Property  Numerator=rxPreambleMFCoeffs  NumeratorPrototype=[]  FilterStructure=Direct form systolic  SerializationOption=Minimum number of cycles between valid input samples  NumCycles=2  NumberOfMultipliers=2  SimulateUsing=Code generation  roundingMode=Floor  overflowMode=off  CoefficientsDataTypeStr=Inherit: Same word length as input  OutputDataTypeStr=Inherit: Same word length as input  ResetInputPort=off  HDLGlobalReset=off  CoeffMultiplier=Multiplier  UseMultForPow2Coeff=on  FrameInputSymmOptim=off
  Magnitude Squared : Subsystem
  Magnitude Squared and Moving Sum : Subsystem
  ThresholdLimiter : MATLAB Function  TreatAsAtomicUnit=on
  dataOut : Outport
  threshold : Outport  Port=2
  validOut : Outport  Port=3
  wires:
  Discrete FIR Filter/2 -> Delay1/1
  validIn/1 -> Magnitude Squared and Moving Sum/2(validIn), Discrete FIR Filter/2
  Discrete FIR Filter/1 -> Delay6/1
  Delay1/1 -> Delay7/1
  Delay3/1 -> validOut/1
  dataIn/1 -> Magnitude Squared and Moving Sum/1(scaled1), Discrete FIR Filter/1
  Delay4/1 -> ThresholdLimiter/1(x)
  Delay2/1 -> dataOut/1
  Delay5/1 -> threshold/1
  Magnitude Squared and Moving Sum/1(E1) -> Delay4/1
  Delay6/1 -> Magnitude Squared/1(In1)
  Magnitude Squared/1(Out1) -> Complex to Real-Imag/1
  ThresholdLimiter/1(y) -> Delay8/1
  Delay7/1 -> Delay3/1
  Delay8/1 -> Delay5/1
  Complex to Real-Imag/1 -> Delay2/1

== system zynqRadioHWSWQPSKAD9361AD9364SL/HDL_QPSK/QPSK Tx Channel QPSK Rx/QPSK Rx/Frequency and Time Synchronizer/Preamble Detector/No HDL ==
  In1 : Inport
  In2 : Inport  Port=2
  Enable : EnablePort
  Correlation Time Scope : Scope  NumInputPorts=2
      settings: TimeUnits=Metric (based on Time Span)  Title=Time Plot of Preamble Detection  ActiveDisplayYMinimum=-0.12629  ActiveDisplayYMaximum=1.13657  YLabel=Amplitude
  Data Type Conversion : DataTypeConversion  OutDataTypeStr=double  SaturateOnIntegerOverflow=off  RndMeth=Floor
  Data Type Conversion1 : DataTypeConversion  OutDataTypeStr=double  SaturateOnIntegerOverflow=off  RndMeth=Floor
  To Workspace : ToWorkspace  VariableName=simPeakFind  SampleTime=-1
      settings: Save2DSignal=2-D array (concatenate along first dimension)
  wires:
  Data Type Conversion1/1 -> Correlation Time Scope/2  "Threshold"
  In2/1 -> Data Type Conversion1/1
  Data Type Conversion/1 -> To Workspace/1, Correlation Time Scope/1  "Correlation Value"
  In1/1 -> Data Type Conversion/1

== system zynqRadioHWSWQPSKAD9361AD9364SL/HDL_QPSK/QPSK Tx Channel QPSK Rx/QPSK Rx/Frequency and Time Synchronizer/Preamble Detector/Peak Search ==
  note: peak picker
  corr : Inport
  thresholdExceeded : Inport  Port=2
  validIn : Inport  Port=3
  Compare To Constant : simulink/Logic and Bit Operations/Compare To Constant  relop===  const=samplesPerFrame1x - 1  OutDataTypeStr=boolean
  Logical Operator : Logic  IconShape=distinctive  AllPortsSameDT=off  OutDataTypeStr=boolean
  Logical Operator4 : Logic  IconShape=distinctive  AllPortsSameDT=off  OutDataTypeStr=boolean
  Relational Operator : RelationalOperator  Operator=>  OutDataTypeStr=boolean  InputSameDT=off
  Terminator : Terminator
  Unit Delay Enabled Synchronous : hdlsllib/Discrete/Unit Delay Enabled Synchronous  InitialCondition=0.0  SampleTime=-1
  Unit Delay Enabled Synchronous1 : hdlsllib/Discrete/Unit Delay Enabled Synchronous  InitialCondition=0.0  SampleTime=-1
  Unit Delay Enabled Resettable Synchronous : hdlsllib/Discrete/Unit Delay Enabled Resettable Synchronous  InitialCondition=0.0  SampleTime=-1
  Unit Delay Enabled Resettable Synchronous1 : hdlsllib/Discrete/Unit Delay Enabled Resettable Synchronous  InitialCondition=0.0  SampleTime=-1
  timing Reference : hdlsllib/Sources/HDL Counter  CountType=Count limited  CountInit=0  CountStep=1  CountMax=samplesPerFrame1x - 1  CountFromType=Initial value  CountFrom=0  CountResetPort=off  CountLoadPort=off  CountEnbPort=on  CountDirPort=off  CountHitOutputPort=off  CountDataType=Unsigned  CountWordLen=nextpow2(samplesPerFrame1x - 1)  CountFracLen=0  CountSampTime=1
  timing Reference Long : hdlsllib/Sources/HDL Counter  CountType=Free running  CountInit=0  CountStep=1  CountMax=samplesPerFrame1x - 1  CountFromType=Initial value  CountFrom=0  CountResetPort=off  CountLoadPort=off  CountEnbPort=on  CountDirPort=off  CountHitOutputPort=off  CountDataType=Unsigned  CountWordLen=32  CountFracLen=0  CountSampTime=1
  timingOffset : Outport
  done : Outport  Port=2
  success : Outport  Port=3
  wires:
  validIn/1 -> Logical Operator/1, timing Reference/1, timing Reference Long/1
  timing Reference Long/1 -> Unit Delay Enabled Synchronous1/1
  timing Reference/1 -> Unit Delay Enabled Synchronous/1, Compare To Constant/1
  thresholdExceeded/1 -> Unit Delay Enabled Resettable Synchronous1/2, Unit Delay Enabled Resettable Synchronous1/1, Logical Operator4/2
  corr/1 -> Unit Delay Enabled Resettable Synchronous/1, Relational Operator/1
  Compare To Constant/1 -> Logical Operator/2
  Logical Operator/1 -> Unit Delay Enabled Resettable Synchronous1/3, done/1, Unit Delay Enabled Resettable Synchronous/3
  Relational Operator/1 -> Logical Operator4/1
  Unit Delay Enabled Resettable Synchronous/1 -> Relational Operator/2
  Unit Delay Enabled Resettable Synchronous1/1 -> success/1
  Logical Operator4/1 -> Unit Delay Enabled Synchronous/2, Unit Delay Enabled Synchronous1/2, Unit Delay Enabled Resettable Synchronous/2
  Unit Delay Enabled Synchronous/1 -> timingOffset/1
  Unit Delay Enabled Synchronous1/1 -> Terminator/1
